simulink model "stellaris_pil_mdlref"  (R2012b)
settings: Solver=FixedStepDiscrete  StartTime=0.0  StopTime=inf  FixedStep=0.1  RelTol=1e-3
settings Model: Creator=peselnikmg  LastModifiedBy=peselnikmg
settings DataIOCC: SignalLoggingSaveFormat=ModelDataLogs  SaveOutput=off  SaveTime=off
settings OptimizationCC: InlineParams=on  OptimizeModelRefInitCode=on  LifeSpan=1
settings HardwareCC: ProdEndianess=LittleEndian  ProdHWDeviceType=Texas Instruments->TMS470
settings RTWCC: SystemTargetFile=stellaris.tlc  TemplateMakefile=stellaris_tmf  PostCodeGenCommand=stellaris_customcode(buildInfo)  Description=TI Stellaris LaunchPad  ProcessScript=stellaris_make_rtw_hook
settings CodeAppCC: IgnoreCustomStorageClasses=off
settings STFCustomTargetCC: CodeReplacementLibrary=ANSI_C  CombineOutputUpdateFcns=on  ERTCustomFileBanners=on  SupportContinuousTime=off  SupportNonInlinedSFcns=off  GRTInterface=off  SystemTargetFile=stellaris.tlc
settings ERTTargetCC: CodeReplacementLibrary=ANSI_C  MultiwordLength=2048  ParMdlRefBuildCompliant=off  CompOptLevelCompliant=off  ConcurrentExecutionCompliant=off  ERTFirstTimeCompliant=off  ModelStepFunctionPrototypeControlCompliant=off  CPPClassGenCompliant=off  InlinedParameterPlacement=NonHierarchical  ERTCustomFileTemplate=stellaris_srmain.tlc  ConvertIfToSwitch=off  SuppressUnreachableDefaultCases=off

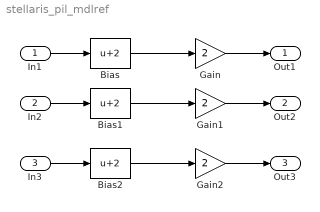
== system stellaris_pil_mdlref ==
  In1 : Inport  OutDataTypeStr=uint8  PortDimensions=1  SampleTime=[0.10000000000000001,0]
  In2 : Inport  Port=2  OutDataTypeStr=uint8  PortDimensions=2  SampleTime=[0.10000000000000001,0]
  In3 : Inport  Port=3  OutDataTypeStr=int32  PortDimensions=2  SampleTime=[0.10000000000000001,0]
  Bias : Bias  Bias=2
  Bias1 : Bias  Bias=2
  Bias2 : Bias  Bias=2
  Gain : Gain  Gain=2  OutDataTypeStr=uint8
  Gain1 : Gain  Gain=2  OutDataTypeStr=uint8
  Gain2 : Gain  Gain=2  OutDataTypeStr=int32
  Out1 : Outport  OutDataTypeStr=uint8  PortDimensions=1  SampleTime=[0.10000000000000001,0]
  Out2 : Outport  Port=2  OutDataTypeStr=uint8  PortDimensions=2  SampleTime=[0.10000000000000001,0]
  Out3 : Outport  Port=3  OutDataTypeStr=int32  PortDimensions=2  SampleTime=[0.10000000000000001,0]
  wires:
  Gain/1 -> Out1/1
  Bias/1 -> Gain/1
  In1/1 -> Bias/1
  Bias1/1 -> Gain1/1
  In2/1 -> Bias1/1
  Gain1/1 -> Out2/1
  Bias2/1 -> Gain2/1
  In3/1 -> Bias2/1
  Gain2/1 -> Out3/1
